simulink model "MAIN_VEHICLE_MODEL"  (R2025b)
settings: Solver=ode4  StartTime=0.0  StopTime=90  FixedStep=0.001  RelTol=1e-3
libraries: rllib x1
settings Model: SimulationMode=accelerator  LastModifiedBy=Gadir
settings SolverCC: AlgebraicLoopSolver=LineSearch
settings DebuggingCC: AlgebraicLoopMsg=none

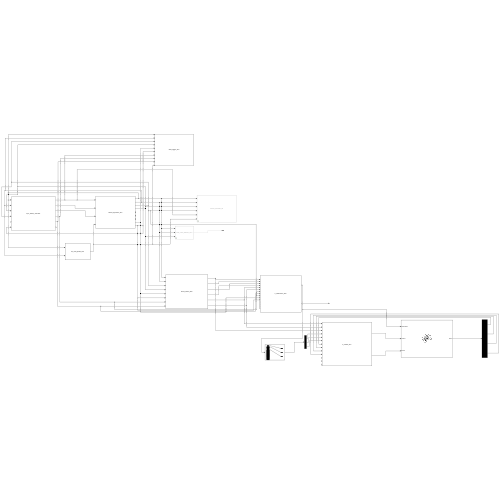
[thumbnail: Simulink's stored preview of the top-level diagram]
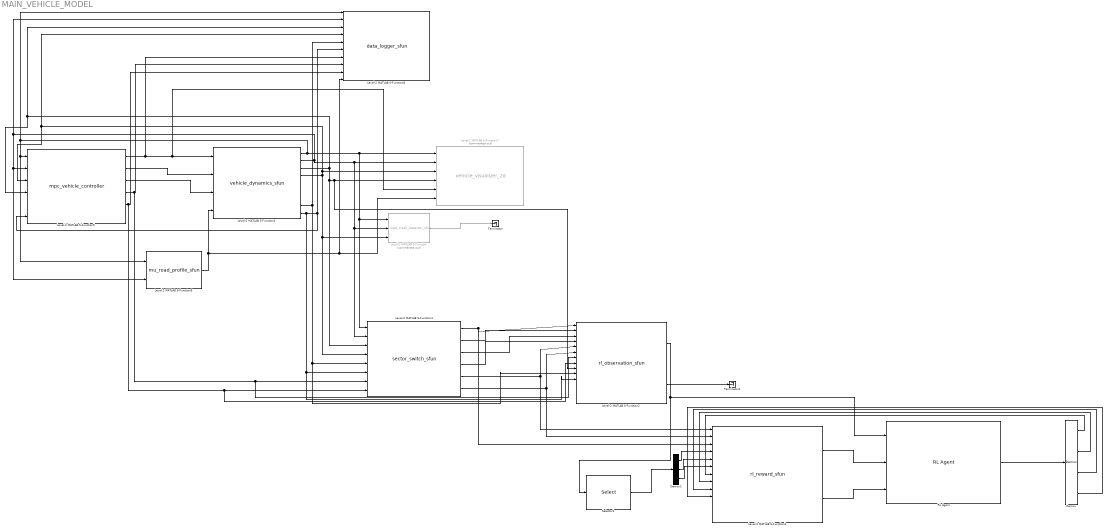
== system MAIN_VEHICLE_MODEL ==
  Demux : Demux
  Demux1 : Demux  Outputs=3
  Level-2 MATLAB S-Function : M-S-Function  Commented=on  FunctionName=road_crash_detector_sfun
  Level-2 MATLAB S-Function1 : M-S-Function  FunctionName=sector_switch_sfun
  Level-2 MATLAB S-Function2 : M-S-Function  FunctionName=rl_observation_sfun
  Level-2 MATLAB S-Function3 : M-S-Function  FunctionName=rl_reward_sfun
  Level-2 MATLAB S-Function4 : M-S-Function  FunctionName=vehicle_dynamics_sfun
  Level-2 MATLAB S-Function5 : M-S-Function  FunctionName=mpc_vehicle_controller
  Level-2 MATLAB S-Function6 : M-S-Function  FunctionName=mu_road_profile_sfun
  Level-2 MATLAB S-Function7 : M-S-Function  Commented=on  FunctionName=vehicle_visualizer_2d
  Level-2 MATLAB S-Function8 : M-S-Function  FunctionName=data_logger_sfun
  RL Agent : rllib/RL Agent  Agent=sac_agent  ExternalActionAsInput=off  ProvideLastAction=off  ProvideCumRwd=off  TreatAsDirectFeedthrough=on  UseStrictObservationDataTypes=off
  Selector1 : Selector  InputPortWidth=16  IndexOptions=Index vector (dialog)  Indices=[1 2 5]  OutputSizes=1
  Terminator : Terminator
  Terminator1 : Terminator
  wires:
  Level-2 MATLAB S-Function5/1 -> Level-2 MATLAB S-Function8/7, Level-2 MATLAB S-Function7/5, Level-2 MATLAB S-Function4/1
  Level-2 MATLAB S-Function5/2 -> Level-2 MATLAB S-Function4/2
  Level-2 MATLAB S-Function5/3 -> Level-2 MATLAB S-Function4/3
  Level-2 MATLAB S-Function6/1 -> Level-2 MATLAB S-Function8/10, Level-2 MATLAB S-Function7/6, Level-2 MATLAB S-Function4/4
  Level-2 MATLAB S-Function4/1 -> Level-2 MATLAB S-Function1/1, Level-2 MATLAB S-Function/1, Level-2 MATLAB S-Function7/1, Level-2 MATLAB S-Function5/1, Level-2 MATLAB S-Function6/1, Level-2 MATLAB S-Function8/1
  Level-2 MATLAB S-Function4/2 -> Level-2 MATLAB S-Function1/2, Level-2 MATLAB S-Function/2, Level-2 MATLAB S-Function7/2, Level-2 MATLAB S-Function8/2, Level-2 MATLAB S-Function6/2, Level-2 MATLAB S-Function5/2
  Level-2 MATLAB S-Function4/4 -> Level-2 MATLAB S-Function1/4, Level-2 MATLAB S-Function/3, Level-2 MATLAB S-Function7/3, Level-2 MATLAB S-Function8/4, Level-2 MATLAB S-Function5/3
  Level-2 MATLAB S-Function4/9 -> Level-2 MATLAB S-Function1/6, Level-2 MATLAB S-Function2/11, Level-2 MATLAB S-Function5/6, Level-2 MATLAB S-Function8/6
  Level-2 MATLAB S-Function4/3 -> Level-2 MATLAB S-Function2/9, Level-2 MATLAB S-Function7/4, Level-2 MATLAB S-Function1/3, Level-2 MATLAB S-Function8/3, Level-2 MATLAB S-Function5/4
  Level-2 MATLAB S-Function4/8 -> Level-2 MATLAB S-Function1/5, Level-2 MATLAB S-Function2/10, Level-2 MATLAB S-Function8/5
  Level-2 MATLAB S-Function5/4 -> Level-2 MATLAB S-Function2/7, Level-2 MATLAB S-Function1/7, Level-2 MATLAB S-Function8/8
  Level-2 MATLAB S-Function5/5 -> Level-2 MATLAB S-Function2/8, Level-2 MATLAB S-Function1/8, Level-2 MATLAB S-Function8/9
  Level-2 MATLAB S-Function/1 -> Terminator/1
  Level-2 MATLAB S-Function1/5 -> Level-2 MATLAB S-Function2/5, Level-2 MATLAB S-Function3/1
  Level-2 MATLAB S-Function1/2 -> Level-2 MATLAB S-Function2/2
  Level-2 MATLAB S-Function1/3 -> Level-2 MATLAB S-Function2/3
  Level-2 MATLAB S-Function1/4 -> Level-2 MATLAB S-Function2/4
  Level-2 MATLAB S-Function1/1 -> Level-2 MATLAB S-Function2/1, Level-2 MATLAB S-Function3/3
  Level-2 MATLAB S-Function1/6 -> Level-2 MATLAB S-Function3/2, Level-2 MATLAB S-Function2/6
  RL Agent/1 -> Demux/1
  Demux/1 -> Level-2 MATLAB S-Function3/7
  Demux/2 -> Level-2 MATLAB S-Function3/8
  Demux/3 -> Level-2 MATLAB S-Function3/9
  Demux/4 -> Level-2 MATLAB S-Function3/10
  Level-2 MATLAB S-Function2/1 -> RL Agent/1, Selector1/1
  Selector1/1 -> Demux1/1
  Demux1/1 -> Level-2 MATLAB S-Function3/4
  Demux1/2 -> Level-2 MATLAB S-Function3/5
  Demux1/3 -> Level-2 MATLAB S-Function3/6
  Level-2 MATLAB S-Function3/1 -> RL Agent/2
  Level-2 MATLAB S-Function3/2 -> RL Agent/3
  Level-2 MATLAB S-Function2/2 -> Terminator1/1
